simulink model "Radar_Nonlinear_model"  (R2020a)
settings: Solver=VariableStepAuto  StartTime=0.0  StopTime=20  RelTol=1e-3
values from neighbouring files (symbols this model uses):
  A = [0, 1, 0, 0, 0, 0 ... (first row only)    [parameters.m]
  B = [0, 0 ... (first row only)    [parameters.m]
  C = [1, 0, 0, 0, 0, 0 ... (first row only)    [parameters.m]
  g = 9.81    [parameters.m]
  Je = 600    [parameters.m]
  K = K_Int(:,1:n)    [parameters.m]    (also in parameters_Int.m)
  Ki = K_Int(:,n+1:end)    [parameters.m]    (also in parameters_Int.m)
  L = place(A',C',des_poles_obsv)'    [parameters.m]
  Le = 0.5    [parameters.m]
  Len_e = sqrt(300)    [parameters.m]
  M_e = 60    [parameters.m]
  r = 0.55    [parameters.m]
  radar_pos = [0;0;0.96]    [parameters.m]
  Re = 1    [parameters.m]
  v = v/8.6603    (= 5.77347205062)    [parameters.m]
  x0 = [0, 0, 0, 0, 0, 0]'    [parameters.m]
  x_r = [pi/6 , 0, 0, pi/4, 0, 0]'    [parameters.m]
  z = z/8.6603    (= 1154.69441012)    [parameters.m]
libraries: vrlib x5
settings Model: Creator=sirius  LastModifiedBy=sirius

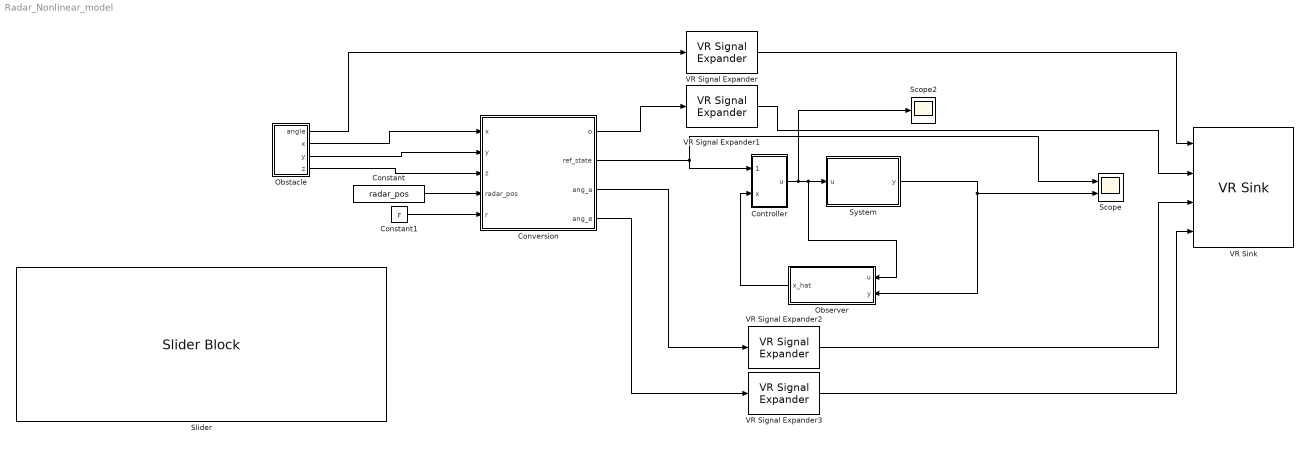
== system Radar_Nonlinear_model ==
  Constant : Constant  Value=radar_pos
  Constant1 : Constant  Value=r
  Controller : Subsystem
  Conversion : MATLAB Function  TreatAsAtomicUnit=on
  Observer : Subsystem
  Obstacle : Subsystem
  Scope : Scope  NumInputPorts=2
  Scope2 : Scope
  Slider : SliderBlock  ScaleMin=-1.5708  ScaleMax=1.5708
  System : Subsystem
  VR Signal Expander : vrlib/VR Signal Expander  outwidth=4  outidx=[4]
  VR Signal Expander1 : vrlib/VR Signal Expander  outwidth=3  outidx=[1 2 3]
  VR Signal Expander2 : vrlib/VR Signal Expander  outwidth=4  outidx=[4]
  VR Signal Expander3 : vrlib/VR Signal Expander  outwidth=4  outidx=[4]
  VR Sink : vrlib/VR Sink  InstantiateOnLoad=on  SampleTime=0.1  ViewEnable=on  RemoteChange=off  RemoteView=off  FieldsWritten=Plane.rotation.4.1.1.double#Plane.translation.3.1.1.double#Axis_1.rotation.4.1.1.double#Axis_2.rotation.4.1.1.double  WorldFileName=Box.wrl  AutoView=off  VideoDimensions=[]  AllowVariableSize=off
  wires:
  Controller/1(u) -> Scope2/1, Observer/1(u), System/1(u)
  System/1(y) -> Observer/2(y), Scope/2
  Observer/1(x_hat) -> Controller/2(x)
  Conversion/2(ref_state) -> Controller/1(ref_state), Scope/1
  Obstacle/2(x) -> Conversion/1(x)
  Obstacle/4(z) -> Conversion/3(z)
  Obstacle/3(y) -> Conversion/2(y)
  Constant/1 -> Conversion/4(radar_pos)
  Constant1/1 -> Conversion/5(r)
  Conversion/1(o) -> VR Signal Expander1/1
  VR Signal Expander1/1 -> VR Sink/2
  Obstacle/1(angle) -> VR Signal Expander/1
  VR Signal Expander/1 -> VR Sink/1
  Conversion/3(ang_a) -> VR Signal Expander2/1
  Conversion/4(ang_e) -> VR Signal Expander3/1
  VR Signal Expander2/1 -> VR Sink/3
  VR Signal Expander3/1 -> VR Sink/4

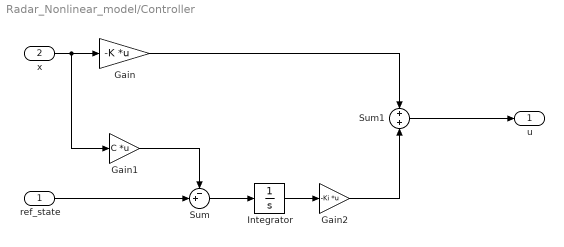
== system Radar_Nonlinear_model/Controller ==
  ref_state : Inport
  x : Inport  Port=2
  Gain : Gain  Gain=-K  Multiplication=Matrix(K*u)
  Gain1 : Gain  Gain=C  Multiplication=Matrix(K*u)
  Gain2 : Gain  Gain=-Ki  Multiplication=Matrix(K*u)
  Integrator : Integrator
  Sum : Sum  Inputs=-+|
  Sum1 : Sum  Inputs=+|+
  u : Outport
  wires:
  x/1 -> Gain1/1, Gain/1
  ref_state/1 -> Sum/2
  Gain1/1 -> Sum/1
  Sum/1 -> Integrator/1
  Integrator/1 -> Gain2/1
  Gain/1 -> Sum1/1
  Gain2/1 -> Sum1/2
  Sum1/1 -> u/1

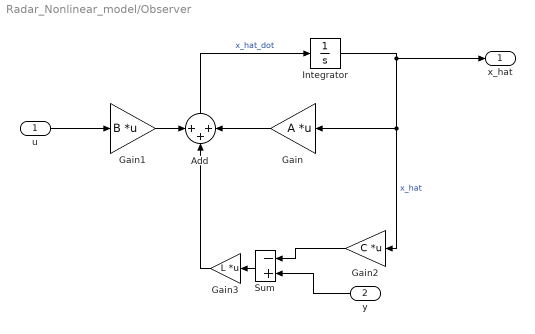
== system Radar_Nonlinear_model/Observer ==
  u : Inport
  y : Inport  Port=2
  Add : Sum  Inputs=+++
  Gain : Gain  Gain=A  Multiplication=Matrix(K*u)
  Gain1 : Gain  Gain=B  Multiplication=Matrix(K*u)
  Gain2 : Gain  Gain=C  Multiplication=Matrix(K*u)
  Gain3 : Gain  Gain=L  Multiplication=Matrix(K*u)
  Integrator : Integrator  InitialCondition=x0  IgnoreLimit=on
  Sum : Sum  Inputs=-+
  x_hat : Outport
  wires:
  Integrator/1 -> x_hat/1, Gain2/1, Gain/1  "x_hat"
  Gain1/1 -> Add/1
  Add/1 -> Integrator/1  "x_hat_dot"
  u/1 -> Gain1/1
  Gain2/1 -> Sum/1
  y/1 -> Sum/2
  Sum/1 -> Gain3/1
  Gain3/1 -> Add/2
  Gain/1 -> Add/3

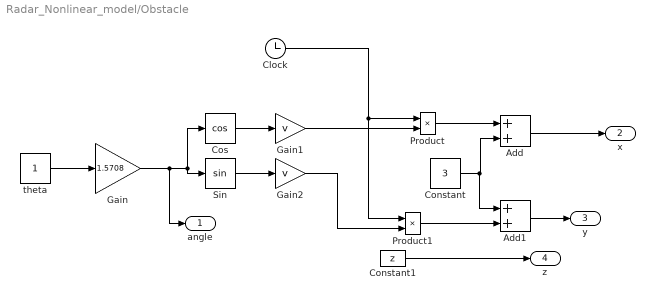
== system Radar_Nonlinear_model/Obstacle ==
  Add : Sum
  Add1 : Sum
  Clock : Clock
  Constant : Constant  Value=3
  Constant1 : Constant  Value=z
  Cos : Trigonometry  Operator=cos
  Gain : Gain  Gain=1.5708
  Gain1 : Gain  Gain=v
  Gain2 : Gain  Gain=v
  Product : Product
  Product1 : Product
  Sin : Trigonometry
  theta : Constant
  angle : Outport
  x : Outport  Port=2
  y : Outport  Port=3
  z : Outport  Port=4
  wires:
  Sin/1 -> Gain2/1
  Gain2/1 -> Product1/2
  Clock/1 -> Product1/1, Product/1
  Cos/1 -> Gain1/1
  Gain/1 -> angle/1, Cos/1, Sin/1
  Constant1/1 -> z/1
  theta/1 -> Gain/1
  Gain1/1 -> Product/2
  Add/1 -> x/1
  Product/1 -> Add/1
  Add1/1 -> y/1
  Product1/1 -> Add1/2
  Constant/1 -> Add1/1, Add/2

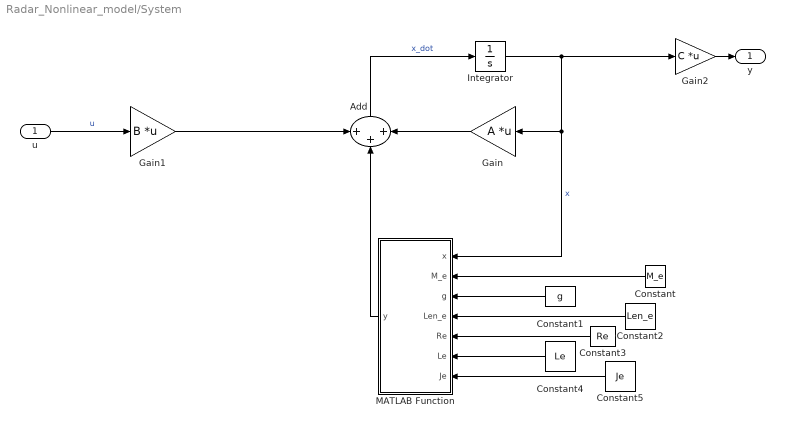
== system Radar_Nonlinear_model/System ==
  u : Inport
  Add : Sum  Inputs=+++
  Constant : Constant  Value=M_e
  Constant1 : Constant  Value=g
  Constant2 : Constant  Value=Len_e
  Constant3 : Constant  Value=Re
  Constant4 : Constant  Value=Le
  Constant5 : Constant  Value=Je
  Gain : Gain  Gain=A  Multiplication=Matrix(K*u)
  Gain1 : Gain  Gain=B  Multiplication=Matrix(K*u)
  Gain2 : Gain  Gain=C  Multiplication=Matrix(K*u)
  Integrator : Integrator  InitialCondition=x_r  IgnoreLimit=on
  MATLAB Function : MATLAB Function  TreatAsAtomicUnit=on
  y : Outport
  wires:
  u/1 -> Gain1/1  "u"
  Constant/1 -> MATLAB Function/2(M_e)
  Constant1/1 -> MATLAB Function/3(g)
  Gain/1 -> Add/3
  Constant5/1 -> MATLAB Function/7(Je)
  Constant2/1 -> MATLAB Function/4(Len_e)
  Constant4/1 -> MATLAB Function/6(Le)
  Integrator/1 -> MATLAB Function/1(x), Gain/1, Gain2/1  "x"
  Add/1 -> Integrator/1  "x_dot"
  Constant3/1 -> MATLAB Function/5(Re)
  MATLAB Function/1(y) -> Add/2
  Gain2/1 -> y/1
  Gain1/1 -> Add/1

== matlab function Radar_Nonlinear_model/Conversion ==
  data: o output; ref_state output; x input; ang_a output; y input; z input; radar_pos input; r input; ang_e output
function [o, ref_state, ang_a , ang_e] = PlaneToAngle(x,y,z,radar_pos,r)

%-------------------------------------------
a1 = x^2 + y^2; b1 = -2*(r^2)*x ; c1 = -(y^2)*r^2 + r^4;
at1 = (-b1 + sqrt(b1^2 - 4*a1*c1))/(2*a1);
at2 = (-b1 - sqrt(b1^2 - 4*a1*c1))/(2*a1);
bt1 = sqrt(r^2 - at1^2);
bt2 = sqrt(r^2 - at2^2);
%-----------------------------------------
t1 = -pi/2 + atan2(-bt1,-at1);
p1x = at1 + cos(t1) ; p1y = bt1 + sin(t1);
d1 = norm([x-p1x, y-p1y]);
t2 = -pi/2 + atan2(-bt2,-at2);
p2x = at2 + cos(t2) ; p2y = bt2 +sin(t2); 
d2 = norm([x-p2x,y-p2y]);
if (d1 <= d2)
    ang_a = -atan2(bt1,at1) ;
else
    ang_a = -atan2(bt2,at2) ;
end
%====================================================
ang_e = atan2(z-radar_pos(3),sqrt(x^2 + y^2));

ref_state = [ang_a; ang_e];
o = [x; z ; -y];

end

== matlab function Radar_Nonlinear_model/System/MATLAB Function ==
  data: x input; y output; M_e input; g input; Len_e input; Re input; Le input; Je input
function y = Nonlinearities(x,M_e,g,Len_e,Re,Le,Je) %x is 6x1 vector
y = [0;
     0;
     0;
     0;
     0;
     (M_e*g*Len_e*Re*sin(x(4))*x(5) - Re*M_e*g*Len_e*cos(x(4)))/(2*Le*Je);
     ];
